simulink library "libbha_bha"  (R2015b)
settings: Solver=FixedStepDiscrete  StartTime=0.0  StopTime=Inf  FixedStep=0.004  RelTol=1e-3
PostLoadFcn:
  | , if any(exist('dsrtsu_mdlpostloadfcn', 'file') == [2, 3, 6]), try dsrtsu_mdlpostloadfcn('Execute', bdroot); catch fprintf('Error in PostLoadFcn (dsrtsu_mdlpostloadfcn) for model "%s":\n %s\n', bdroot, lasterr); end, end,
undefined symbols (not defined in the file or in its folder): accurate, BHA, O
libraries: libbha_io x7, libc_filters_diff x6, libbha_kinematic_tools x6, rtilibm x4, libbha_bha x1, libc_extended_basics x1
settings Model: DSRTSU_INTERNAL_RTI_VER=470  DSRTSU_INTERNAL_RTI_TYPE=rti1007  DSRTSU_INTERNAL_RTIFPGA=60  Creator=Falkenhahn  LastModifiedBy=isysfalkenhahn
settings DataIOCC: SaveFormat=Array
settings OptimizationCC: BlockReduction=off  OptimizeBlockIOStorage=off  BufferReuse=off  GlobalBufferReuse=off  ExpressionFolding=off  LocalBlockOutputs=off
settings DebuggingCC: UnderspecifiedInitializationDetection=Classic  MergeDetectMultiDrivingBlocksExec=none  SolverPrmCheckMsg=warning
settings HardwareCC: ProdBitPerPointer=32  ProdLargestAtomicFloat=None  ProdEndianess=BigEndian  ProdWordSize=32  ProdHWDeviceType=Generic->Custom  TargetIntDivRoundTo=Zero  TargetEndianess=BigEndian  TargetHWDeviceType=Generic->Custom
settings RTWCC: SystemTargetFile=rti1007.tlc  MakeCommand=make_rti  TemplateMakefile=rti1007.tmf  Description=dSPACE DS1007 Hardware Platform
settings STFCustomTargetCC: ParMdlRefBuildCompliant=on  ConcurrentExecutionCompliant=off  MatFileLogging=on  SystemTargetFile=rti1007.tlc
settings GRTTargetCC: CompOptLevelCompliant=off  ConcurrentExecutionCompliant=off  GeneratePreprocessorConditionals=Disable all  CombineOutputUpdateFcns=off  GRTInterface=on  UseToolchainInfoCompliant=off  ExtModeMexFile=noextcomm
settings ConfigComp: CovModelRefEnable=Off

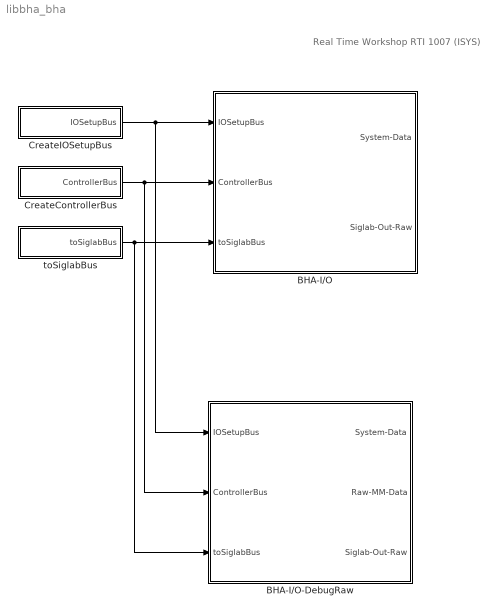
== system libbha_bha ==
  note: Real Time Workshop
      | RTI 1007 (ISYS)
  BHA-I/O : Subsystem  mask{tA=0.001 % CONST.tA, tA_mm=0.001 % CTRL.Measurement.tA, tA_mm_CAN=0.001 % CTRL.Measurement.tA_CAN, f_length=24 % CTRL.Measurement.f_filt_length, f_pressure=25 % 50 % CTRL.Measurement.f_filt_pressure, f_raw=0.1 % CTRL.Measurement.f_filt_raw}
      mask prompts: tA "simulation sample time [s]"; tA_mm "measurement sample time [s]"; tA_mm_CAN "measurement sample time (CAN) [s]"; f_length "filter frequency length [Hz]"; f_pressure "filter frequency pressure [Hz]"; f_raw "filter frequency raw [Hz]"
      settings: AttributesFormatString=|
      | simulation sample time: %<tA>
      | mm sample time: %<tA_mm>
      | mm sample time (CAN): %<tA_mm_CAN>
      | filter length: %<f_length> Hz
      | filter pressure: %<f_pressure> Hz
      | filter raw: %<f_raw> Hz
  BHA-I/O-DebugRaw : Subsystem  mask{tA=0.001 % CONST.tA, tA_mm=0.001 % CTRL.Measurement.tA, tA_mm_CAN=0.004 % CTRL.Measurement.tA_CAN, f_length=24 % CTRL.Measurement.f_filt_length, f_pressure=24 % 50 % CTRL.Measurement.f_filt_pressure, f_raw=0.1 % CTRL.Measurement.f_filt_raw}
      mask prompts: tA "simulation sample time [s]"; tA_mm "measurement sample time [s]"; tA_mm_CAN "measurement sample time (CAN) [s]"; f_length "filter frequency length [Hz]"; f_pressure "filter frequency pressure [Hz]"; f_raw "filter frequency raw [Hz]"
      settings: AttributesFormatString=|
      | simulation sample time: %<tA>
      | mm sample time: %<tA_mm>
      | mm sample time (CAN): %<tA_mm_CAN>
      | filter length: %<f_length> Hz
      | filter pressure: %<f_pressure> Hz
      | filter raw: %<f_raw> Hz
  CreateControllerBus : Subsystem
  CreateIOSetupBus : Subsystem
  toSiglabBus : Subsystem
  wires:
  CreateIOSetupBus/1(IOSetupBus) -> BHA-I/O/1(IOSetupBus), BHA-I/O-DebugRaw/1(IOSetupBus)
  CreateControllerBus/1(ControllerBus) -> BHA-I/O/2(ControllerBus), BHA-I/O-DebugRaw/2(ControllerBus)
  toSiglabBus/1(toSiglabBus) -> BHA-I/O/3(toSiglabBus), BHA-I/O-DebugRaw/3(toSiglabBus)

== system libbha_bha/BHA-I//O ==
  note: Real Time Workshop
      | RTI 1007 (ISYS)
  IOSetupBus : Inport
  ControllerBus : Inport  Port=2
  toSiglabBus : Inport  Port=3
  BHA-I/O-DebugRaw : libbha_bha/BHA-I//O-DebugRaw  tA=tA  tA_mm=tA_mm  tA_mm_CAN=tA_mm_CAN  f_length=f_length  f_pressure=f_pressure  f_raw=f_raw
      settings: AttributesFormatString=|
      | simulation sample time: %<tA>
      | mm sample time: %<tA_mm>
      | mm sample time (CAN): %<tA_mm_CAN>
      | filter length: %<f_length> Hz
      | filter pressure: %<f_pressure> Hz
      | filter raw: %<f_raw> Hz
  Terminator : Terminator
  System-Data : Outport
  Siglab-Out-Raw : Outport  Port=2
  wires:
  BHA-I/O-DebugRaw/1 -> System-Data/1
  BHA-I/O-DebugRaw/3 -> Siglab-Out-Raw/1
  toSiglabBus/1 -> BHA-I/O-DebugRaw/3
  ControllerBus/1 -> BHA-I/O-DebugRaw/2
  IOSetupBus/1 -> BHA-I/O-DebugRaw/1
  BHA-I/O-DebugRaw/2 -> Terminator/1

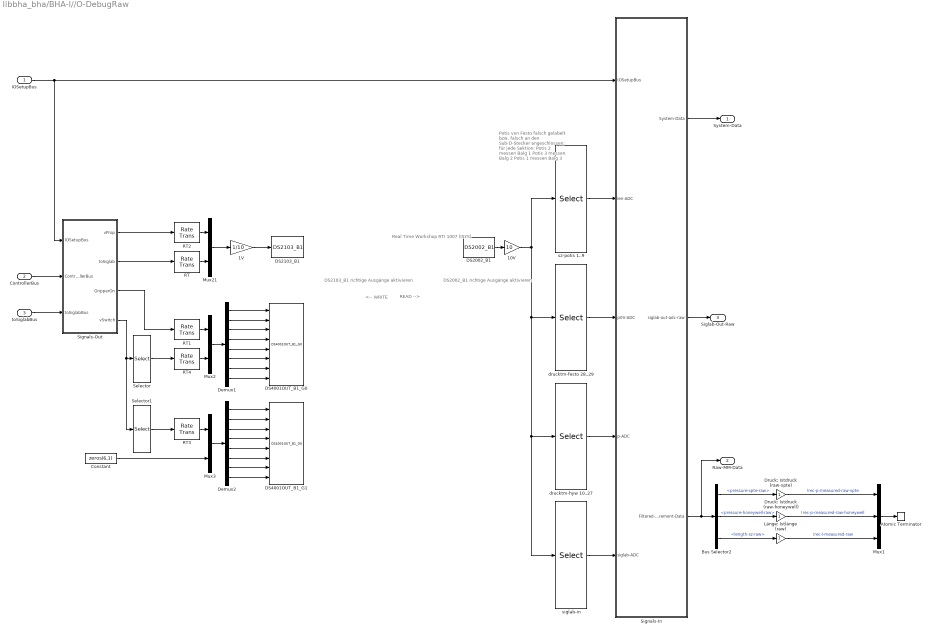
== system libbha_bha/BHA-I//O-DebugRaw ==
  note: Potis von Festo falsch
      | gelabelt bzw. falsch an
      | den Sub-D-Stecker
      | angeschlossen:
      | für jede Sektion:
      | Potis 2 messen Balg 1
      | Potis 3 messen Balg 2
      | Potis 1 messen Balg 3
  note: DS2103_B1 richtige Ausgänge aktivieren
  note: DS2002_B1 richtige Ausgänge aktivieren
  note: <-- WRITE
  note: READ -->
  note: Real Time Workshop
      | RTI 1007 (ISYS)
  IOSetupBus : Inport
  ControllerBus : Inport  Port=2
  toSiglabBus : Inport  Port=3
  10V : Gain  Gain=10
  1V : Gain  Gain=1/10
  Atomic Terminator : libc_extended_basics/Atomic Terminator
  Bus Selector2 : BusSelector  OutputSignals=pressure-spte-raw,pressure-honeywell-raw,length-sz-raw
  Constant : Constant  Value=zeros(6,1)  OutDataTypeStr=boolean
  DS2002_B1 : rtilibm/DS2002/DS2002_B1  BoardNo=1  ChannelNos=[1 2 3 4 5 6 7 8 9 10 11 12 13 14 15 16 17 18 19 20 21 22 23 24 25 26 27 28 29 30 31 32]  Range=[10 10]  Resolution=[16 16]  SampleAndHoldMode=[1 1]  DialogFcn=gui2002  UnitName={ 'DS2002_B' }  UnitValues={ 1 }  DSProperties=struct('RTI',struct('Version',uint32(1),'BlockType',struct('isSLSource',uint8(1),'isSLSink',uint8(0),'isHWSource',uint8(1),'isHWSink',uint8(0),'isSetup',uint8(0),'isInline',uint8(1),'isNonInline',uint8(0),'isInterrupt',uint8(0),'isChannelwise',uint8(0)),'IOBoardType','DS2002','UnitType','ADC','Identifier','ADCMUX','DialogType','ML','BlockSet','NONE','SlaveProcessor','NONE'))
  DS2103_B1 : rtilibm/DS2103/DS2103_B1  BoardNo=1  ChannelNos=[1 2 3 4 5 6 7 8 9 10 11 12]  Range=[10 10 10 10 10 10 10 10 10 10 10 10 10 10 10 10 10 10 10 10 10 10 10 10 10 10 10 10 10 10 10 10]  IOErrorMode=[1 1 1 1 1 1 1 1]  InitValue=[0.5 0.5 0.5 0.5 0.5 0.5 0.5 0.5 0 0 0 0 0 0 0 0 0 0 0 0 0 0 0 0 0 0 0 0 0 0 0 0]  TermMode=[0 0 0 0 0 0 0 0 1 1 1 1 1 1 1 1 1 1 1 1 1 1 1 1 1 1 1 1 1 1 1 1]  TermValue=[0 0 0 0 0 0 0 0 0 0 0 0 0 0 0 0 0 0 0 0 0 0 0 0 0 0 0 0 0 0 0 0]  DialogFcn=gui2103  UnitName={ 'DS2103_B' }  UnitValues={ 1 }  DSProperties=struct('RTI',struct('Version',uint32(1),'BlockType',struct('isSLSource',uint8(0),'isSLSink',uint8(1),'isHWSource',uint8(0),'isHWSink',uint8(1),'isSetup',uint8(0),'isInline',uint8(1),'isNonInline',uint8(0),'isInterrupt',uint8(0),'isChannelwise',uint8(0)),'IOBoardType','DS2103','UnitType','DAC','Identifier','DACMUX','DialogType','ML','BlockSet','NONE','SlaveProcessor','NONE'))
  DS4001OUT_B1_G0 : rtilibm/DS4001/DS4001OUT_B1_G0  BoardNo=1  GroupNo=0  InitValue=[0 0 0 0 0 0 0 0]  TermMode=[1 1 1 1 1 1 1 1]  TermValue=[0 0 0 0 0 0 0 0]  DialogFcn=gui400xout  UnitName={ 'DS4001OUT_B', '_G' }  UnitValues="{ 1  0 }"  DSProperties=struct('RTI',struct('Version',uint32(1),'BlockType',struct('isSLSource',uint8(0),'isSLSink',uint8(1),'isHWSource',uint8(0),'isHWSink',uint8(1),'isSetup',uint8(0),'isInline',uint8(1),'isNonInline',uint8(0),'isInterrupt',uint8(0),'isChannelwise',uint8(0)),'IOBoardType','DS4001','UnitType','BIT','Identifier','BITOUT','DialogType','ML','BlockSet','NONE','SlaveProcessor','NONE'))
  DS4001OUT_B1_G1 : rtilibm/DS4001/DS4001OUT_B1_G0  BoardNo=1  GroupNo=1  InitValue=[0 0 0 0 0 0 0 0]  TermMode=[1 1 1 1 1 1 1 1]  TermValue=[0 0 0 0 0 0 0 0]  DialogFcn=gui400xout  UnitName={ 'DS4001OUT_B', '_G' }  UnitValues="{1  1}"  DSProperties=struct('RTI',struct('Version',uint32(1),'BlockType',struct('isSLSource',uint8(0),'isSLSink',uint8(1),'isHWSource',uint8(0),'isHWSink',uint8(1),'isSetup',uint8(0),'isInline',uint8(1),'isNonInline',uint8(0),'isInterrupt',uint8(0),'isChannelwise',uint8(0)),'IOBoardType','DS4001','UnitType','BIT','Identifier','BITOUT','DialogType','ML','BlockSet','NONE','SlaveProcessor','NONE'))
  Demux1 : Demux  Outputs=8
  Demux2 : Demux  Outputs=8
  Druck: Istdruck (raw-honeywell) : Gain
  Druck: Istdruck (raw-spte) : Gain
  Länge: Istlänge (raw) : Gain
  Mux1 : Mux  Inputs=3
  Mux2 : Mux  Inputs=2
  Mux21 : Mux  Inputs=2
  Mux3 : Mux  Inputs=2
  RT{,1..4} (5 alike) : RateTransition  Deterministic=off  OutPortSampleTime=tA_mm
  Selector : Selector  InputPortWidth=9  IndexOptions=Index vector (dialog)  Indices=[1 2 3 4 5 6 7]  OutputSizes=1
  Selector1 : Selector  InputPortWidth=9  IndexOptions=Index vector (dialog)  Indices=[8 9]  OutputSizes=1
  Signals-In : Subsystem
      settings: AttributesFormatString=|
      | sample time: tA
      | (simulation sample time)
  Signals-Out : Subsystem
  drucktm-festo 28..29 : Selector  InputPortWidth=32  IndexOptions=Index vector (dialog)  Indices=[28 29]  OutputSizes=1
  "drucktm-hyw 10..27 " : Selector  InputPortWidth=32  IndexOptions=Index vector (dialog)  Indices=[10 11 12 13 14 15 16 17 18 19 20 21 22 23 24 25 26 27]  OutputSizes=1
  siglab-in : Selector  InputPortWidth=32  IndexOptions=Index vector (dialog)  Indices=[30 31 32]  OutputSizes=1
  sz-potis 1..9 : Selector  InputPortWidth=32  IndexOptions=Index vector (dialog)  Indices=[2 3 1 5 6 4 8 9 7]  OutputSizes=1
  System-Data : Outport
  Raw-MM-Data : Outport  Port=2
  Siglab-Out-Raw : Outport  Port=3
  wires:
  RT3/1 -> Mux3/1
  Mux3/1 -> Demux2/1
  RT4/1 -> Mux2/2
  RT1/1 -> Mux2/1
  Mux2/1 -> Demux1/1
  Bus Selector2/2 -> Druck: Istdruck (raw-honeywell)/1  "<pressure-honeywell-raw>"
  Bus Selector2/3 -> Länge: Istlänge (raw)/1  "<length-sz-raw>"
  Druck: Istdruck (raw-honeywell)/1 -> Mux1/2  "!rec-p-measured-raw-honeywell"
  Länge: Istlänge (raw)/1 -> Mux1/3  "!rec-l-measured-raw"
  Mux1/1 -> Atomic Terminator/1
  Signals-In/1(System-Data) -> System-Data/1
  toSiglabBus/1 -> Signals-Out/3(toSiglabBus)
  IOSetupBus/1 -> Signals-In/1(IOSetupBus), Signals-Out/1(IOSetupBus)
  ControllerBus/1 -> Signals-Out/2(ControllerBus)
  Signals-Out/2(toSiglab) -> RT/1
  Signals-Out/1(vProp) -> RT2/1
  1V/1 -> DS2103_B1/1
  10V/1 -> siglab-in/1, "drucktm-hyw 10..27 "/1, drucktm-festo 28..29/1, sz-potis 1..9/1
  DS2002_B1/1 -> 10V/1
  Mux21/1 -> 1V/1
  RT2/1 -> Mux21/1
  RT/1 -> Mux21/2
  Demux1/2 -> DS4001OUT_B1_G0/2
  Demux1/6 -> DS4001OUT_B1_G0/6
  Demux1/1 -> DS4001OUT_B1_G0/1
  Demux1/3 -> DS4001OUT_B1_G0/3
  Demux1/5 -> DS4001OUT_B1_G0/5
  Demux1/8 -> DS4001OUT_B1_G0/8
  Demux1/4 -> DS4001OUT_B1_G0/4
  Demux1/7 -> DS4001OUT_B1_G0/7
  Demux2/3 -> DS4001OUT_B1_G1/3
  Demux2/1 -> DS4001OUT_B1_G1/1
  Demux2/4 -> DS4001OUT_B1_G1/4
  Demux2/2 -> DS4001OUT_B1_G1/2
  Demux2/5 -> DS4001OUT_B1_G1/5
  Demux2/6 -> DS4001OUT_B1_G1/6
  Demux2/7 -> DS4001OUT_B1_G1/7
  Demux2/8 -> DS4001OUT_B1_G1/8
  Signals-Out/4(vSwitch) -> Selector1/1, Selector/1
  Signals-Out/3(GripperOn) -> RT1/1
  Selector/1 -> RT4/1
  Selector1/1 -> RT3/1
  Constant/1 -> Mux3/2
  sz-potis 1..9/1 -> Signals-In/2(len-ADC)
  drucktm-festo 28..29/1 -> Signals-In/3(p0V-ADC)
  siglab-in/1 -> Signals-In/5(siglab-ADC)
  "drucktm-hyw 10..27 "/1 -> Signals-In/4(p-ADC)
  Signals-In/3(Filtered-Raw-Measurement-Data) -> Bus Selector2/1, Raw-MM-Data/1
  Signals-In/2(siglab-out-adc-raw) -> Siglab-Out-Raw/1
  Bus Selector2/1 -> Druck: Istdruck (raw-spte)/1  "<pressure-spte-raw>"
  Druck: Istdruck (raw-spte)/1 -> Mux1/1  "!rec-p-measured-raw-spte"

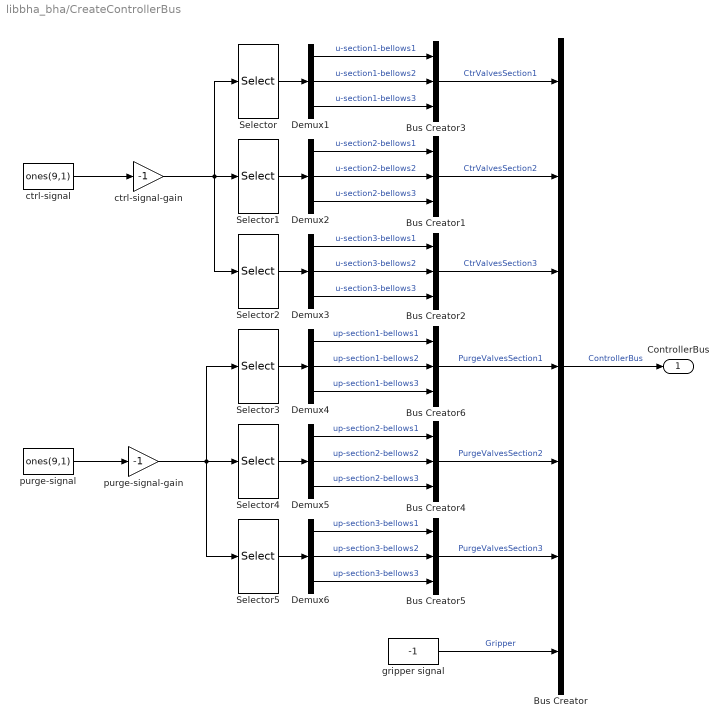
== system libbha_bha/CreateControllerBus ==
  Bus Creator : BusCreator  Inputs=7
  Bus Creator{1..6} (6 alike) : BusCreator  Inputs=3
  Demux{1..6} (6 alike) : Demux  Outputs=3
  Selector : Selector  InputPortWidth=9  IndexOptions=Index vector (dialog)  Indices=[1 2 3]  OutputSizes=1
  Selector1 : Selector  InputPortWidth=9  IndexOptions=Index vector (dialog)  Indices=[4 5 6]  OutputSizes=1
  Selector2 : Selector  InputPortWidth=9  IndexOptions=Index vector (dialog)  Indices=[7 8 9]  OutputSizes=1
  Selector3 : Selector  InputPortWidth=9  IndexOptions=Index vector (dialog)  Indices=[1 2 3]  OutputSizes=1
  Selector4 : Selector  InputPortWidth=9  IndexOptions=Index vector (dialog)  Indices=[4 5 6]  OutputSizes=1
  Selector5 : Selector  InputPortWidth=9  IndexOptions=Index vector (dialog)  Indices=[7 8 9]  OutputSizes=1
  ctrl-signal : Constant  Value=ones(9,1)
  ctrl-signal-gain : Gain  Gain=-1
  gripper signal : Constant  Value=-1
  purge-signal : Constant  Value=ones(9,1)
  purge-signal-gain : Gain  Gain=-1
  ControllerBus : Outport
  wires:
  Demux3/3 -> Bus Creator2/3  "u-section3-bellows3"
  Demux3/2 -> Bus Creator2/2  "u-section3-bellows2"
  Demux3/1 -> Bus Creator2/1  "u-section3-bellows1"
  Demux2/1 -> Bus Creator1/1  "u-section2-bellows1"
  Demux2/2 -> Bus Creator1/2  "u-section2-bellows2"
  Demux2/3 -> Bus Creator1/3  "u-section2-bellows3"
  Demux1/1 -> Bus Creator3/1  "u-section1-bellows1"
  Demux1/2 -> Bus Creator3/2  "u-section1-bellows2"
  Demux1/3 -> Bus Creator3/3  "u-section1-bellows3"
  Bus Creator/1 -> ControllerBus/1  "ControllerBus"
  Selector/1 -> Demux1/1
  Selector1/1 -> Demux2/1
  Selector2/1 -> Demux3/1
  Bus Creator3/1 -> Bus Creator/1  "CtrValvesSection1"
  Bus Creator1/1 -> Bus Creator/2  "CtrValvesSection2"
  Bus Creator2/1 -> Bus Creator/3  "CtrValvesSection3"
  Demux6/3 -> Bus Creator5/3  "up-section3-bellows3"
  Demux6/2 -> Bus Creator5/2  "up-section3-bellows2"
  Demux6/1 -> Bus Creator5/1  "up-section3-bellows1"
  Demux5/1 -> Bus Creator4/1  "up-section2-bellows1"
  Demux5/2 -> Bus Creator4/2  "up-section2-bellows2"
  Demux5/3 -> Bus Creator4/3  "up-section2-bellows3"
  Demux4/1 -> Bus Creator6/1  "up-section1-bellows1"
  Demux4/2 -> Bus Creator6/2  "up-section1-bellows2"
  Demux4/3 -> Bus Creator6/3  "up-section1-bellows3"
  Selector3/1 -> Demux4/1
  Selector4/1 -> Demux5/1
  Selector5/1 -> Demux6/1
  Bus Creator6/1 -> Bus Creator/4  "PurgeValvesSection1"
  Bus Creator4/1 -> Bus Creator/5  "PurgeValvesSection2"
  Bus Creator5/1 -> Bus Creator/6  "PurgeValvesSection3"
  ctrl-signal/1 -> ctrl-signal-gain/1
  purge-signal/1 -> purge-signal-gain/1
  purge-signal-gain/1 -> Selector5/1, Selector3/1, Selector4/1
  ctrl-signal-gain/1 -> Selector2/1, Selector/1, Selector1/1
  gripper signal/1 -> Bus Creator/7  "Gripper"

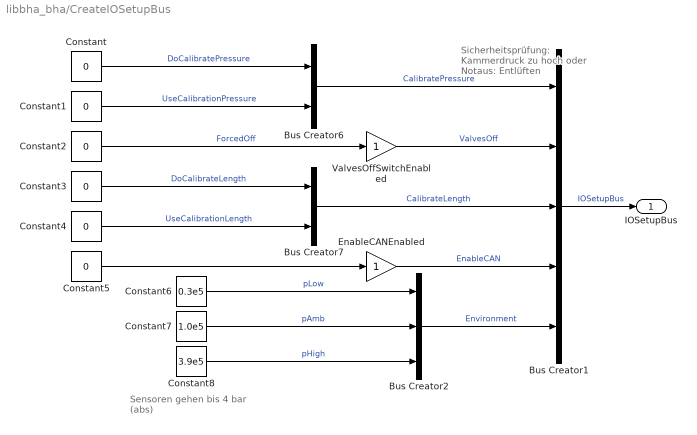
== system libbha_bha/CreateIOSetupBus ==
  note: Sensoren gehen bis 4 bar (abs)
  note: Sicherheitsprüfung:
      | Kammerdruck zu hoch
      | oder Notaus: Entlüften
  Bus Creator1 : BusCreator  Inputs=5
  Bus Creator2 : BusCreator  Inputs=3
  Bus Creator6 : BusCreator  Inputs=2
  Bus Creator7 : BusCreator  Inputs=2
  Constant{,1..5} (6 alike) : Constant  Value=0
  Constant6 : Constant  Value=0.3e5
  Constant7 : Constant  Value=1.0e5
  Constant8 : Constant  Value=3.9e5
  EnableCANEnabled : Gain
  ValvesOffSwitchEnabled : Gain
  IOSetupBus : Outport
  wires:
  Constant8/1 -> Bus Creator2/3  "pHigh"
  Constant7/1 -> Bus Creator2/2  "pAmb"
  Constant6/1 -> Bus Creator2/1  "pLow"
  Bus Creator1/1 -> IOSetupBus/1  "IOSetupBus"
  Bus Creator7/1 -> Bus Creator1/3  "CalibrateLength"
  Constant/1 -> Bus Creator6/1  "DoCalibratePressure"
  Constant1/1 -> Bus Creator6/2  "UseCalibrationPressure"
  Constant3/1 -> Bus Creator7/1  "DoCalibrateLength"
  Constant4/1 -> Bus Creator7/2  "UseCalibrationLength"
  Bus Creator2/1 -> Bus Creator1/5  "Environment"
  ValvesOffSwitchEnabled/1 -> Bus Creator1/2  "ValvesOff"
  Bus Creator6/1 -> Bus Creator1/1  "CalibratePressure"
  Constant5/1 -> EnableCANEnabled/1
  EnableCANEnabled/1 -> Bus Creator1/4  "EnableCAN"
  Constant2/1 -> ValvesOffSwitchEnabled/1  "ForcedOff"

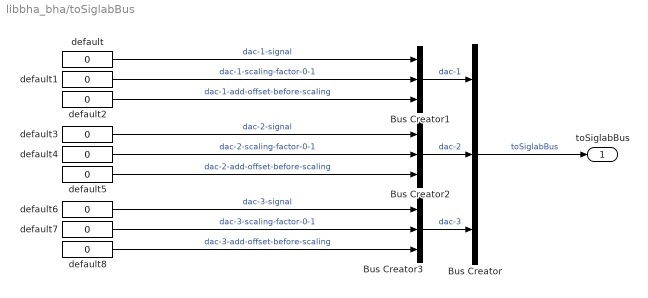
== system libbha_bha/toSiglabBus ==
  Bus Creator{,1..3} (4 alike) : BusCreator  Inputs=3
  default{,1..8} (9 alike) : Constant  Value=0
  toSiglabBus : Outport
  wires:
  default6/1 -> Bus Creator3/1  "dac-3-signal"
  default7/1 -> Bus Creator3/2  "dac-3-scaling-factor-0-1"
  default8/1 -> Bus Creator3/3  "dac-3-add-offset-before-scaling"
  default3/1 -> Bus Creator2/1  "dac-2-signal"
  default4/1 -> Bus Creator2/2  "dac-2-scaling-factor-0-1"
  default5/1 -> Bus Creator2/3  "dac-2-add-offset-before-scaling"
  default2/1 -> Bus Creator1/3  "dac-1-add-offset-before-scaling"
  default/1 -> Bus Creator1/1  "dac-1-signal"
  default1/1 -> Bus Creator1/2  "dac-1-scaling-factor-0-1"
  Bus Creator3/1 -> Bus Creator/3  "dac-3"
  Bus Creator2/1 -> Bus Creator/2  "dac-2"
  Bus Creator1/1 -> Bus Creator/1  "dac-1"
  Bus Creator/1 -> toSiglabBus/1  "toSiglabBus"

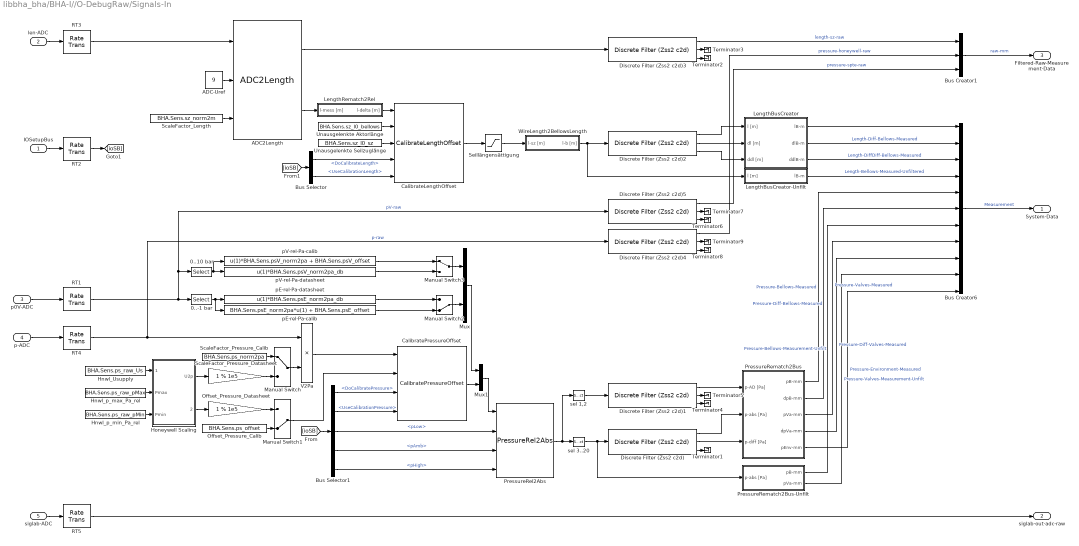
== system libbha_bha/BHA-I//O-DebugRaw/Signals-In ==
  IOSetupBus : Inport
  len-ADC : Inport  Port=2
  p0V-ADC : Inport  Port=3
  p-ADC : Inport  Port=4
      settings: AttributesFormatString=|
      | 1..9 pValves (a)
      | 10..18 pBellows (b)
  siglab-ADC : Inport  Port=5
  0..-1 bar : Selector  InputPortWidth=2  IndexOptions=Index vector (dialog)  Indices=1  OutputSizes=1
      settings: AttributesFormatString=0..10 V
  0..10 bar : Selector  InputPortWidth=2  IndexOptions=Index vector (dialog)  Indices=2  OutputSizes=1
      settings: AttributesFormatString=0..10 V
  ADC-Uref : Constant  Value=9
  ADC2Length : libbha_io/ADC2Length
  Bus Creator1 : BusCreator  Inputs=3
  Bus Creator6 : BusCreator  Inputs=11
  Bus Selector : BusSelector  OutputSignals=CalibrateLength.DoCalibrateLength,CalibrateLength.UseCalibrationLength
  Bus Selector1 : BusSelector  OutputSignals=CalibratePressure.DoCalibratePressure,CalibratePressure.UseCalibrationPressure,Environment.pLow,Environment.pAmb,Environment.pHigh
  CalibrateLengthOffset : libbha_io/CalibrateLengthOffset
  CalibratePressureOffset : libbha_io/CalibratePressureOffset
      settings: AttributesFormatString=Dimension: %<dim>
  Discrete Filter (Zss2 c2d) : libc_filters_diff/Discrete Filter (Zss2 c2d)  rdnname2342_gf=f_pressure  rdnname2342_tA=tA  rdnname2342_mode=noh (d=0)  rdnname2342_diffmode=O(2) [accurate]  rdnname2342_showd=on
      settings: AttributesFormatString=%<rdnname2342_gf> Hz, %<rdnname2342_mode>
  Discrete Filter (Zss2 c2d)1 : libc_filters_diff/Discrete Filter (Zss2 c2d)  rdnname2342_gf=f_pressure  rdnname2342_tA=tA  rdnname2342_mode=noh (d=0)  rdnname2342_diffmode=O(2) [accurate]  rdnname2342_showd=on
      settings: AttributesFormatString=%<rdnname2342_gf> Hz, %<rdnname2342_mode>
  Discrete Filter (Zss2 c2d)2 : libc_filters_diff/Discrete Filter (Zss2 c2d)  rdnname2342_gf=f_length  rdnname2342_tA=tA  rdnname2342_mode=noh (d=0)  rdnname2342_diffmode=O(2) [accurate]  rdnname2342_showd=on
      settings: AttributesFormatString=%<rdnname2342_gf> Hz, %<rdnname2342_mode>
  Discrete Filter (Zss2 c2d)3 : libc_filters_diff/Discrete Filter (Zss2 c2d)  rdnname2342_gf=f_raw  rdnname2342_tA=tA  rdnname2342_mode=zoh (d=dt)  rdnname2342_diffmode=O(2) [accurate]  rdnname2342_showd=on
      settings: AttributesFormatString=%<rdnname2342_gf> Hz, %<rdnname2342_mode>
  Discrete Filter (Zss2 c2d)4 : libc_filters_diff/Discrete Filter (Zss2 c2d)  rdnname2342_gf=f_raw  rdnname2342_tA=tA  rdnname2342_mode=zoh (d=dt)  rdnname2342_diffmode=O(2) [accurate]  rdnname2342_showd=on
      settings: AttributesFormatString=%<rdnname2342_gf> Hz, %<rdnname2342_mode>
  Discrete Filter (Zss2 c2d)5 : libc_filters_diff/Discrete Filter (Zss2 c2d)  rdnname2342_gf=f_raw  rdnname2342_tA=tA  rdnname2342_mode=zoh (d=dt)  rdnname2342_diffmode=O(2) [accurate]  rdnname2342_showd=on
      settings: AttributesFormatString=%<rdnname2342_gf> Hz, %<rdnname2342_mode>
  Hnwl_Usupply : Constant  Value=BHA.Sens.ps_raw_Us
  Hnwl_p_max_Pa_rel : Constant  Value=BHA.Sens.ps_raw_pMax
  Hnwl_p_min_Pa_rel : Constant  Value=BHA.Sens.ps_raw_pMin
  Honeywell Scaling : MATLAB Function  TreatAsAtomicUnit=on
  LengthBusCreator : Subsystem
  LengthBusCreator-Unfilt : Subsystem
  LengthRematch2Rel : Subsystem
  Manual Switch : ManualSwitch
  Manual Switch1 : ManualSwitch  CurrentSetting=0
  Manual Switch2 : ManualSwitch  CurrentSetting=0
  Manual Switch3 : ManualSwitch
  Mux : Mux  Inputs=2
  Mux1 : Mux  Inputs=2
  Offset_Pressure_Calib : Constant  Value=BHA.Sens.ps_offset
  Offset_Pressure_Datasheet : Gain  Gain=1 % 1e5
  PressureRel2Abs : libbha_io/PressureRel2Abs
  PressureRematch2Bus : Subsystem
  PressureRematch2Bus-Unfilt : Subsystem
  RT1 : RateTransition  Deterministic=off  X0=1.1  OutPortSampleTime=tA
      settings: AttributesFormatString=|
      | sinnv. Anfangswert:
      | 1.1
  RT2 : RateTransition  Deterministic=off  OutPortSampleTime=tA
  RT3 : RateTransition  Deterministic=off  X0=[3 3 3 4 4 4 5 5 5]  OutPortSampleTime=tA
      settings: AttributesFormatString=|
      | sinnv. Anfangswerte:
      | [ 3 3 3 4 4 4 5 5 5 ]
  RT4 : RateTransition  Deterministic=off  X0=5  OutPortSampleTime=tA
      settings: AttributesFormatString=|
      | sinnv. Anfangswert:
      | 5
  RT5 : RateTransition  Deterministic=off  OutPortSampleTime=tA
  ScaleFactor_Length : Constant  Value=BHA.Sens.sz_norm2m
  ScaleFactor_Pressure_Calib : Constant  Value=BHA.Sens.ps_norm2pa
  ScaleFactor_Pressure_Datasheet : Gain  Gain=1 % 1e5
  Seillängensättigung : Saturate  UpperLimit=2.0  LowerLimit=0.1
      settings: AttributesFormatString=0.1 bis 2.0
  Terminator{1..9} (9 alike) : Terminator
  Unausgelenkte Aktorlänge : Constant  Value=BHA.Sens.sz_l0_bellows
  Unausgelenkte Seilzuglänge : Constant  Value=BHA.Sens.sz_l0_sz
  V2Pa : Product
  WireLength2BellowsLength : Subsystem
  pE-rel-Pa-calib : Fcn  Expr=BHA.Sens.psE_norm2pa*u(1) + BHA.Sens.psE_offset
  pE-rel-Pa-datasheet : Fcn  Expr=u(1)*BHA.Sens.psE_norm2pa_db
  pV-rel-Pa-calib : Fcn  Expr=u(1)*BHA.Sens.psV_norm2pa + BHA.Sens.psV_offset
  pV-rel-Pa-datasheet : Fcn  Expr=u(1)*BHA.Sens.psV_norm2pa_db
  sel 1,2 : Selector  InputPortWidth=20  IndexOptions=Index vector (dialog)  Indices=[1 2]  OutputSizes=1
  sel 3..20 : Selector  InputPortWidth=20  IndexOptions=Starting index (dialog)  Indices=3  OutputSizes=18
  System-Data : Outport
  siglab-out-adc-raw : Outport  Port=2
  Filtered-Raw-Measurement-Data : Outport  Port=3
  wires:
  Offset_Pressure_Calib/1 -> Manual Switch1/2
  ScaleFactor_Pressure_Calib/1 -> Manual Switch/1
  Offset_Pressure_Datasheet/1 -> Manual Switch1/1
  ScaleFactor_Pressure_Datasheet/1 -> Manual Switch/2
  pE-rel-Pa-datasheet/1 -> Manual Switch2/1
  pV-rel-Pa-datasheet/1 -> Manual Switch3/2
  0..-1 bar/1 -> pE-rel-Pa-calib/1, pE-rel-Pa-datasheet/1
  0..10 bar/1 -> pV-rel-Pa-calib/1, pV-rel-Pa-datasheet/1
  Manual Switch1/1 -> CalibratePressureOffset/2
  Manual Switch/1 -> V2Pa/2
  Honeywell Scaling/2(offset_p) -> Offset_Pressure_Datasheet/1
  Honeywell Scaling/1(U2p) -> ScaleFactor_Pressure_Datasheet/1
  Hnwl_p_min_Pa_rel/1 -> Honeywell Scaling/3(Pmin)
  Hnwl_p_max_Pa_rel/1 -> Honeywell Scaling/2(Pmax)
  Hnwl_Usupply/1 -> Honeywell Scaling/1(Vsupply)
  Bus Creator1/1 -> Filtered-Raw-Measurement-Data/1  "raw-mm"
  Discrete Filter (Zss2 c2d)4/1 -> Bus Creator1/2  "pressure-honeywell-raw"
  Discrete Filter (Zss2 c2d)5/1 -> Bus Creator1/3  "pressure-spte-raw"
  Discrete Filter (Zss2 c2d)4/3 -> Terminator8/1
  Discrete Filter (Zss2 c2d)4/2 -> Terminator9/1
  Discrete Filter (Zss2 c2d)5/3 -> Terminator6/1
  Discrete Filter (Zss2 c2d)5/2 -> Terminator7/1
  Discrete Filter (Zss2 c2d)3/3 -> Terminator2/1
  Discrete Filter (Zss2 c2d)3/2 -> Terminator3/1
  Discrete Filter (Zss2 c2d)3/1 -> Bus Creator1/1  "length-sz-raw"
  PressureRematch2Bus/4(dpVa-mm) -> Bus Creator6/9  "Pressure-Diff-Valves-Measured"
  PressureRematch2Bus/3(pVa-mm) -> Bus Creator6/8  "Pressure-Valves-Measured"
  PressureRematch2Bus-Unfilt/2(pVa-mm) -> Bus Creator6/10  "Pressure-Valves-Measurement-Unfilt"
  LengthBusCreator/1(lB-m) -> Bus Creator6/1
  PressureRematch2Bus-Unfilt/1(pB-mm) -> Bus Creator6/7  "Pressure-Bellows-Measurement-Unfilt"
  LengthBusCreator-Unfilt/1(lB-m) -> Bus Creator6/4  "Length-Bellows-Measured-Unfiltered"
  LengthBusCreator/3(ddlB-m) -> Bus Creator6/3  "Length-DiffDiff-Bellows-Measured"
  LengthBusCreator/2(dlB-m) -> Bus Creator6/2  "Length-Diff-Bellows-Measured"
  PressureRematch2Bus/2(dpB-mm) -> Bus Creator6/6  "Pressure-Diff-Bellows-Measured"
  PressureRematch2Bus/5(pEnv-mm) -> Bus Creator6/11  "Pressure-Environment-Measured"
  PressureRematch2Bus/1(pB-mm) -> Bus Creator6/5  "Pressure-Bellows-Measured"
  Bus Creator6/1 -> System-Data/1  "Measurement"
  Discrete Filter (Zss2 c2d)1/1 -> PressureRematch2Bus/1(p-AD [Pa])
  Discrete Filter (Zss2 c2d)/1 -> PressureRematch2Bus/2(p-abs [Pa])
  Discrete Filter (Zss2 c2d)/2 -> PressureRematch2Bus/3(p-diff [Pa])
  Discrete Filter (Zss2 c2d)/3 -> Terminator1/1
  Discrete Filter (Zss2 c2d)1/3 -> Terminator4/1
  Discrete Filter (Zss2 c2d)1/2 -> Terminator5/1
  Discrete Filter (Zss2 c2d)2/3 -> LengthBusCreator/3(ddl [m])
  Discrete Filter (Zss2 c2d)2/2 -> LengthBusCreator/2(dl [m])
  Discrete Filter (Zss2 c2d)2/1 -> LengthBusCreator/1(l [m])
  sel 1,2/1 -> Discrete Filter (Zss2 c2d)1/1
  sel 3..20/1 -> Discrete Filter (Zss2 c2d)/1, PressureRematch2Bus-Unfilt/1(p-abs [Pa])
  RT5/1 -> siglab-out-adc-raw/1
  PressureRel2Abs/1 -> sel 1,2/1, sel 3..20/1
  WireLength2BellowsLength/1(l-b [m]) -> Discrete Filter (Zss2 c2d)2/1, LengthBusCreator-Unfilt/1(l [m])
  ScaleFactor_Length/1 -> ADC2Length/3
  CalibratePressureOffset/1 -> Mux1/2
  V2Pa/1 -> CalibratePressureOffset/1
  Bus Selector1/1 -> CalibratePressureOffset/3  "<DoCalibratePressure>"
  ADC2Length/1 -> Discrete Filter (Zss2 c2d)3/1
  RT4/1 -> V2Pa/1, Discrete Filter (Zss2 c2d)4/1  "p-raw"
  RT1/1 -> Discrete Filter (Zss2 c2d)5/1, 0..10 bar/1, 0..-1 bar/1  "pV-raw"
  RT3/1 -> ADC2Length/1
  ADC-Uref/1 -> ADC2Length/2
  RT2/1 -> [ioSB]
  siglab-ADC/1 -> RT5/1
  IOSetupBus/1 -> RT2/1
  Mux/1 -> Mux1/1
  p0V-ADC/1 -> RT1/1
  Mux1/1 -> PressureRel2Abs/1
  p-ADC/1 -> RT4/1
  Bus Selector1/5 -> PressureRel2Abs/4  "<pHigh>"
  Bus Selector1/4 -> PressureRel2Abs/3  "<pAmb>"
  Bus Selector1/3 -> PressureRel2Abs/2  "<pLow>"
  Bus Selector1/2 -> CalibratePressureOffset/4  "<UseCalibrationPressure>"
  [ioSB] -> Bus Selector1/1
  len-ADC/1 -> RT3/1
  Bus Selector/2 -> CalibrateLengthOffset/5  "<UseCalibrationLength>"
  Bus Selector/1 -> CalibrateLengthOffset/4  "<DoCalibrateLength>"
  [ioSB] -> Bus Selector/1
  pE-rel-Pa-calib/1 -> Manual Switch2/2
  pV-rel-Pa-calib/1 -> Manual Switch3/1
  Manual Switch3/1 -> Mux/1
  Manual Switch2/1 -> Mux/2
  ADC2Length/2 -> LengthRematch2Rel/1("l-mess [m] ")
  CalibrateLengthOffset/1 -> Seillängensättigung/1
  Unausgelenkte Seilzuglänge/1 -> CalibrateLengthOffset/3
  Unausgelenkte Aktorlänge/1 -> CalibrateLengthOffset/2
  LengthRematch2Rel/1(l-delta [m]) -> CalibrateLengthOffset/1
  Seillängensättigung/1 -> WireLength2BellowsLength/1(l-sz [m])

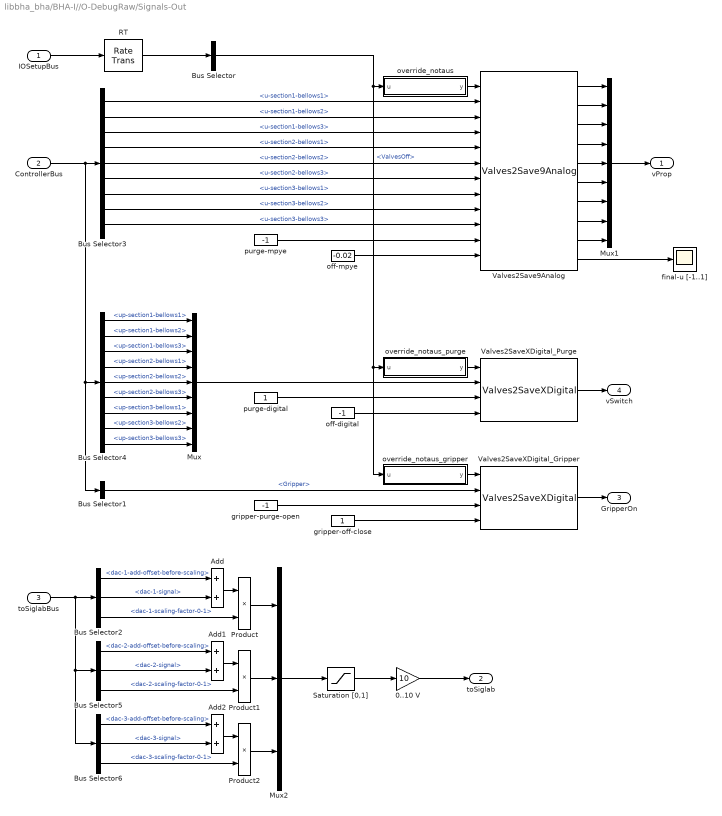
== system libbha_bha/BHA-I//O-DebugRaw/Signals-Out ==
  IOSetupBus : Inport
  ControllerBus : Inport  Port=2
  toSiglabBus : Inport  Port=3
  0..10 V : Gain  Gain=10
  Add : Sum
  Add1 : Sum
  Add2 : Sum
  Bus Selector : BusSelector  OutputSignals=ValvesOff
  Bus Selector1 : BusSelector  OutputSignals=Gripper
  Bus Selector2 : BusSelector  OutputSignals=dac-1.dac-1-add-offset-before-scaling,dac-1.dac-1-signal,dac-1.dac-1-scaling-factor-0-1
  Bus Selector3 : BusSelector  OutputSignals=CtrValvesSection1.u-section1-bellows1,CtrValvesSection1.u-section1-bellows2,CtrValvesSection1.u-section1-bellows3,CtrValvesSection2.u-section2-bellows1,CtrValvesSection2.u-section2-bellows2,CtrValvesSection2.u-section2-bellows3,CtrValvesSection3.u-section3-bellows1,CtrValvesSection3.u-section3-bellows2,CtrValvesSection3.u-section3-bellows3
  Bus Selector4 : BusSelector  OutputSignals=PurgeValvesSection1.up-section1-bellows1,PurgeValvesSection1.up-section1-bellows2,PurgeValvesSection1.up-section1-bellows3,PurgeValvesSection2.up-section2-bellows1,PurgeValvesSection2.up-section2-bellows2,PurgeValvesSection2.up-section2-bellows3,PurgeValvesSection3.up-section3-bellows1,PurgeValvesSection3.up-section3-bellows2,PurgeValvesSection3.up-section3-bellows3
  Bus Selector5 : BusSelector  OutputSignals=dac-2.dac-2-add-offset-before-scaling,dac-2.dac-2-signal,dac-2.dac-2-scaling-factor-0-1
  Bus Selector6 : BusSelector  OutputSignals=dac-3.dac-3-add-offset-before-scaling,dac-3.dac-3-signal,dac-3.dac-3-scaling-factor-0-1
  Mux : Mux  Inputs=9
  Mux1 : Mux  Inputs=9
  Mux2 : Mux  Inputs=3
  Product : Product
  Product1 : Product
  Product2 : Product
  RT : RateTransition  Deterministic=off
  Saturation [0,1] : Saturate  UpperLimit=1  LowerLimit=0
  Valves2Save9Analog : libbha_io/Valves2Save9Analog
  Valves2SaveXDigital_Gripper : libbha_io/Valves2SaveXDigital
  Valves2SaveXDigital_Purge : libbha_io/Valves2SaveXDigital
  final-u [-1..1] : Scope
  gripper-off-close : Constant
  gripper-purge-open : Constant  Value=-1
  off-digital : Constant  Value=-1
  off-mpye : Constant  Value=-0.02
  override_notaus : MATLAB Function  TreatAsAtomicUnit=on
  override_notaus_gripper : MATLAB Function  TreatAsAtomicUnit=on
  override_notaus_purge : MATLAB Function  TreatAsAtomicUnit=on
  purge-digital : Constant
  purge-mpye : Constant  Value=-1
  vProp : Outport
  toSiglab : Outport  Port=2
  GripperOn : Outport  Port=3
  vSwitch : Outport  Port=4
  wires:
  Add/1 -> Product/1
  Bus Selector2/3 -> Product/2  "<dac-1-scaling-factor-0-1>"
  Bus Selector2/2 -> Add/2  "<dac-1-signal>"
  Bus Selector2/1 -> Add/1  "<dac-1-add-offset-before-scaling>"
  0..10 V/1 -> toSiglab/1
  RT/1 -> Bus Selector/1
  Saturation [0,1]/1 -> 0..10 V/1
  Bus Selector/1 -> override_notaus_gripper/1(u), override_notaus_purge/1(u), override_notaus/1(u)  "<ValvesOff>"
  off-mpye/1 -> Valves2Save9Analog/12
  purge-mpye/1 -> Valves2Save9Analog/11
  Valves2Save9Analog/10 -> final-u [-1..1]/1
  IOSetupBus/1 -> RT/1
  Valves2Save9Analog/1 -> Mux1/1
  Valves2Save9Analog/2 -> Mux1/2
  Valves2Save9Analog/3 -> Mux1/3
  Valves2Save9Analog/4 -> Mux1/4
  Valves2Save9Analog/5 -> Mux1/5
  Valves2Save9Analog/6 -> Mux1/6
  Valves2Save9Analog/7 -> Mux1/7
  Valves2Save9Analog/8 -> Mux1/8
  Valves2Save9Analog/9 -> Mux1/9
  Mux1/1 -> vProp/1
  Bus Selector3/9 -> Valves2Save9Analog/10  "<u-section3-bellows3>"
  Bus Selector3/8 -> Valves2Save9Analog/9  "<u-section3-bellows2>"
  Bus Selector3/7 -> Valves2Save9Analog/8  "<u-section3-bellows1>"
  Bus Selector3/6 -> Valves2Save9Analog/7  "<u-section2-bellows3>"
  Bus Selector3/5 -> Valves2Save9Analog/6  "<u-section2-bellows2>"
  Bus Selector3/4 -> Valves2Save9Analog/5  "<u-section2-bellows1>"
  Bus Selector3/3 -> Valves2Save9Analog/4  "<u-section1-bellows3>"
  Bus Selector3/2 -> Valves2Save9Analog/3  "<u-section1-bellows2>"
  Bus Selector3/1 -> Valves2Save9Analog/2  "<u-section1-bellows1>"
  Bus Selector4/1 -> Mux/1  "<up-section1-bellows1>"
  Bus Selector4/2 -> Mux/2  "<up-section1-bellows2>"
  Bus Selector4/3 -> Mux/3  "<up-section1-bellows3>"
  Bus Selector4/4 -> Mux/4  "<up-section2-bellows1>"
  Bus Selector4/5 -> Mux/5  "<up-section2-bellows2>"
  ControllerBus/1 -> Bus Selector4/1, Bus Selector1/1, Bus Selector3/1
  Bus Selector4/6 -> Mux/6  "<up-section2-bellows3>"
  Bus Selector4/7 -> Mux/7  "<up-section3-bellows1>"
  Bus Selector4/8 -> Mux/8  "<up-section3-bellows2>"
  Bus Selector4/9 -> Mux/9  "<up-section3-bellows3>"
  purge-digital/1 -> Valves2SaveXDigital_Purge/3
  off-digital/1 -> Valves2SaveXDigital_Purge/4
  Mux/1 -> Valves2SaveXDigital_Purge/2
  Valves2SaveXDigital_Purge/1 -> vSwitch/1
  Add1/1 -> Product1/1
  Bus Selector5/3 -> Product1/2  "<dac-2-scaling-factor-0-1>"
  Bus Selector5/2 -> Add1/2  "<dac-2-signal>"
  Bus Selector5/1 -> Add1/1  "<dac-2-add-offset-before-scaling>"
  Add2/1 -> Product2/1
  Bus Selector6/3 -> Product2/2  "<dac-3-scaling-factor-0-1>"
  Bus Selector6/2 -> Add2/2  "<dac-3-signal>"
  Bus Selector6/1 -> Add2/1  "<dac-3-add-offset-before-scaling>"
  toSiglabBus/1 -> Bus Selector2/1, Bus Selector5/1, Bus Selector6/1
  Product2/1 -> Mux2/3
  Product1/1 -> Mux2/2
  Product/1 -> Mux2/1
  Mux2/1 -> Saturation [0,1]/1
  Valves2SaveXDigital_Gripper/1 -> GripperOn/1
  gripper-purge-open/1 -> Valves2SaveXDigital_Gripper/3
  gripper-off-close/1 -> Valves2SaveXDigital_Gripper/4
  Bus Selector1/1 -> Valves2SaveXDigital_Gripper/2  "<Gripper>"
  override_notaus_purge/1(y) -> Valves2SaveXDigital_Purge/1
  override_notaus/1(y) -> Valves2Save9Analog/1
  override_notaus_gripper/1(y) -> Valves2SaveXDigital_Gripper/1

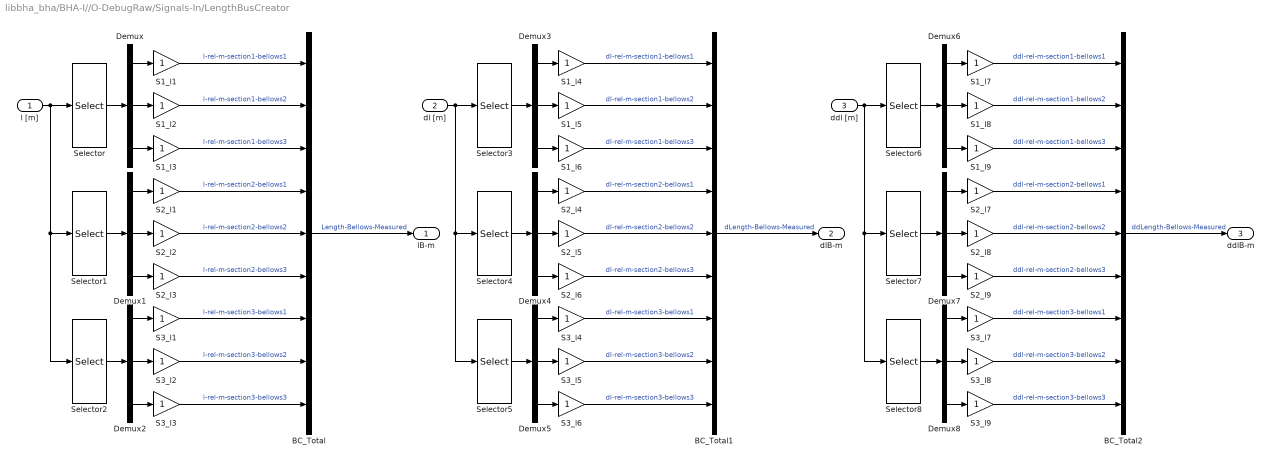
== system libbha_bha/BHA-I//O-DebugRaw/Signals-In/LengthBusCreator ==
  l [m] : Inport
  dl [m] : Inport  Port=2
  ddl [m] : Inport  Port=3
  BC_Total : BusCreator  Inputs=9
  BC_Total1 : BusCreator  Inputs=9
  BC_Total2 : BusCreator  Inputs=9
  Demux{,1..8} (9 alike) : Demux  Outputs=3
  S1_l{1..9} (9 alike) : Gain
  S2_l{1..9} (9 alike) : Gain
  S3_l{1..9} (9 alike) : Gain
  Selector : Selector  InputPortWidth=9  IndexOptions=Index vector (dialog)  Indices=[1 2 3]  OutputSizes=1
  Selector1 : Selector  InputPortWidth=9  IndexOptions=Index vector (dialog)  Indices=[4 5 6]  OutputSizes=1
  Selector2 : Selector  InputPortWidth=9  IndexOptions=Index vector (dialog)  Indices=[7 8 9]  OutputSizes=1
  Selector3 : Selector  InputPortWidth=9  IndexOptions=Index vector (dialog)  Indices=[1 2 3]  OutputSizes=1
  Selector4 : Selector  InputPortWidth=9  IndexOptions=Index vector (dialog)  Indices=[4 5 6]  OutputSizes=1
  Selector5 : Selector  InputPortWidth=9  IndexOptions=Index vector (dialog)  Indices=[7 8 9]  OutputSizes=1
  Selector6 : Selector  InputPortWidth=9  IndexOptions=Index vector (dialog)  Indices=[1 2 3]  OutputSizes=1
  Selector7 : Selector  InputPortWidth=9  IndexOptions=Index vector (dialog)  Indices=[4 5 6]  OutputSizes=1
  Selector8 : Selector  InputPortWidth=9  IndexOptions=Index vector (dialog)  Indices=[7 8 9]  OutputSizes=1
  lB-m : Outport
  dlB-m : Outport  Port=2
  ddlB-m : Outport  Port=3
  wires:
  BC_Total/1 -> lB-m/1  "Length-Bellows-Measured"
  S3_l1/1 -> BC_Total/7  "l-rel-m-section3-bellows1"
  S1_l2/1 -> BC_Total/2  "l-rel-m-section1-bellows2"
  S1_l3/1 -> BC_Total/3  "l-rel-m-section1-bellows3"
  S2_l1/1 -> BC_Total/4  "l-rel-m-section2-bellows1"
  S3_l2/1 -> BC_Total/8  "l-rel-m-section3-bellows2"
  S3_l3/1 -> BC_Total/9  "l-rel-m-section3-bellows3"
  S2_l2/1 -> BC_Total/5  "l-rel-m-section2-bellows2"
  S2_l3/1 -> BC_Total/6  "l-rel-m-section2-bellows3"
  S1_l1/1 -> BC_Total/1  "l-rel-m-section1-bellows1"
  Demux/1 -> S1_l1/1
  Demux/2 -> S1_l2/1
  Demux/3 -> S1_l3/1
  Demux1/2 -> S2_l2/1
  Demux1/1 -> S2_l1/1
  Demux1/3 -> S2_l3/1
  Demux2/1 -> S3_l1/1
  Demux2/2 -> S3_l2/1
  Demux2/3 -> S3_l3/1
  Selector/1 -> Demux/1
  Selector1/1 -> Demux1/1
  Selector2/1 -> Demux2/1
  l [m]/1 -> Selector2/1, Selector1/1, Selector/1
  BC_Total1/1 -> dlB-m/1  "dLength-Bellows-Measured"
  S3_l4/1 -> BC_Total1/7  "dl-rel-m-section3-bellows1"
  S1_l5/1 -> BC_Total1/2  "dl-rel-m-section1-bellows2"
  S1_l6/1 -> BC_Total1/3  "dl-rel-m-section1-bellows3"
  S2_l4/1 -> BC_Total1/4  "dl-rel-m-section2-bellows1"
  S3_l5/1 -> BC_Total1/8  "dl-rel-m-section3-bellows2"
  S3_l6/1 -> BC_Total1/9  "dl-rel-m-section3-bellows3"
  S2_l5/1 -> BC_Total1/5  "dl-rel-m-section2-bellows2"
  S2_l6/1 -> BC_Total1/6  "dl-rel-m-section2-bellows3"
  S1_l4/1 -> BC_Total1/1  "dl-rel-m-section1-bellows1"
  Demux3/1 -> S1_l4/1
  Demux3/2 -> S1_l5/1
  Demux3/3 -> S1_l6/1
  Demux4/2 -> S2_l5/1
  Demux4/1 -> S2_l4/1
  Demux4/3 -> S2_l6/1
  Demux5/1 -> S3_l4/1
  Demux5/2 -> S3_l5/1
  Demux5/3 -> S3_l6/1
  Selector3/1 -> Demux3/1
  Selector4/1 -> Demux4/1
  Selector5/1 -> Demux5/1
  dl [m]/1 -> Selector3/1, Selector4/1, Selector5/1
  BC_Total2/1 -> ddlB-m/1  "ddLength-Bellows-Measured"
  S3_l7/1 -> BC_Total2/7  "ddl-rel-m-section3-bellows1"
  S1_l8/1 -> BC_Total2/2  "ddl-rel-m-section1-bellows2"
  S1_l9/1 -> BC_Total2/3  "ddl-rel-m-section1-bellows3"
  S2_l7/1 -> BC_Total2/4  "ddl-rel-m-section2-bellows1"
  S3_l8/1 -> BC_Total2/8  "ddl-rel-m-section3-bellows2"
  S3_l9/1 -> BC_Total2/9  "ddl-rel-m-section3-bellows3"
  S2_l8/1 -> BC_Total2/5  "ddl-rel-m-section2-bellows2"
  S2_l9/1 -> BC_Total2/6  "ddl-rel-m-section2-bellows3"
  S1_l7/1 -> BC_Total2/1  "ddl-rel-m-section1-bellows1"
  Demux6/1 -> S1_l7/1
  Demux6/2 -> S1_l8/1
  Demux6/3 -> S1_l9/1
  Demux7/2 -> S2_l8/1
  Demux7/1 -> S2_l7/1
  Demux7/3 -> S2_l9/1
  Demux8/1 -> S3_l7/1
  Demux8/2 -> S3_l8/1
  Demux8/3 -> S3_l9/1
  Selector6/1 -> Demux6/1
  Selector7/1 -> Demux7/1
  Selector8/1 -> Demux8/1
  ddl [m]/1 -> Selector8/1, Selector7/1, Selector6/1

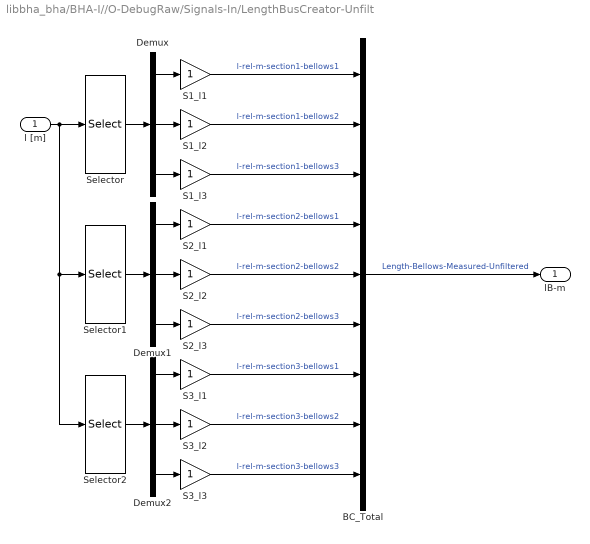
== system libbha_bha/BHA-I//O-DebugRaw/Signals-In/LengthBusCreator-Unfilt ==
  l [m] : Inport
  BC_Total : BusCreator  Inputs=9
  Demux : Demux  Outputs=3
  Demux1 : Demux  Outputs=3
  Demux2 : Demux  Outputs=3
  S1_l1 : Gain
  S1_l2 : Gain
  S1_l3 : Gain
  S2_l1 : Gain
  S2_l2 : Gain
  S2_l3 : Gain
  S3_l1 : Gain
  S3_l2 : Gain
  S3_l3 : Gain
  Selector : Selector  InputPortWidth=9  IndexOptions=Index vector (dialog)  Indices=[1 2 3]  OutputSizes=1
  Selector1 : Selector  InputPortWidth=9  IndexOptions=Index vector (dialog)  Indices=[4 5 6]  OutputSizes=1
  Selector2 : Selector  InputPortWidth=9  IndexOptions=Index vector (dialog)  Indices=[7 8 9]  OutputSizes=1
  lB-m : Outport
  wires:
  l [m]/1 -> Selector/1, Selector1/1, Selector2/1
  Selector2/1 -> Demux2/1
  Selector1/1 -> Demux1/1
  Selector/1 -> Demux/1
  Demux2/3 -> S3_l3/1
  Demux2/2 -> S3_l2/1
  Demux2/1 -> S3_l1/1
  Demux1/3 -> S2_l3/1
  Demux1/1 -> S2_l1/1
  Demux1/2 -> S2_l2/1
  Demux/3 -> S1_l3/1
  Demux/2 -> S1_l2/1
  Demux/1 -> S1_l1/1
  S1_l1/1 -> BC_Total/1  "l-rel-m-section1-bellows1"
  S2_l3/1 -> BC_Total/6  "l-rel-m-section2-bellows3"
  S2_l2/1 -> BC_Total/5  "l-rel-m-section2-bellows2"
  S3_l3/1 -> BC_Total/9  "l-rel-m-section3-bellows3"
  S3_l2/1 -> BC_Total/8  "l-rel-m-section3-bellows2"
  S2_l1/1 -> BC_Total/4  "l-rel-m-section2-bellows1"
  S1_l3/1 -> BC_Total/3  "l-rel-m-section1-bellows3"
  S1_l2/1 -> BC_Total/2  "l-rel-m-section1-bellows2"
  S3_l1/1 -> BC_Total/7  "l-rel-m-section3-bellows1"
  BC_Total/1 -> lB-m/1  "Length-Bellows-Measured-Unfiltered"

== system libbha_bha/BHA-I//O-DebugRaw/Signals-In/LengthRematch2Rel ==
  "l-mess [m] " : Inport
  Demux : Demux  Outputs=9
  Mux : Mux  Inputs=9
  Sum{,1..5} (6 alike) : Sum  Inputs=-+|
  l-delta [m] : Outport
  wires:
  Mux/1 -> l-delta [m]/1
  "l-mess [m] "/1 -> Demux/1
  Demux/1 -> Sum/1, Mux/1  "Bellows1"
  Demux/2 -> Sum1/1, Mux/2  "Bellows2"
  Demux/3 -> Sum2/1, Mux/3  "Bellows3"
  Demux/4 -> Sum/2, Sum3/1
  Demux/5 -> Sum1/2, Sum4/1
  Demux/6 -> Sum2/2, Sum5/1
  Demux/7 -> Sum3/2
  Demux/8 -> Sum4/2
  Demux/9 -> Sum5/2
  Sum/1 -> Mux/4  "Bellows1"
  Sum1/1 -> Mux/5  "Bellows2"
  Sum2/1 -> Mux/6  "Bellows3"
  Sum3/1 -> Mux/7  "Bellows1"
  Sum4/1 -> Mux/8  "Bellows2"
  Sum5/1 -> Mux/9  "Bellows3"

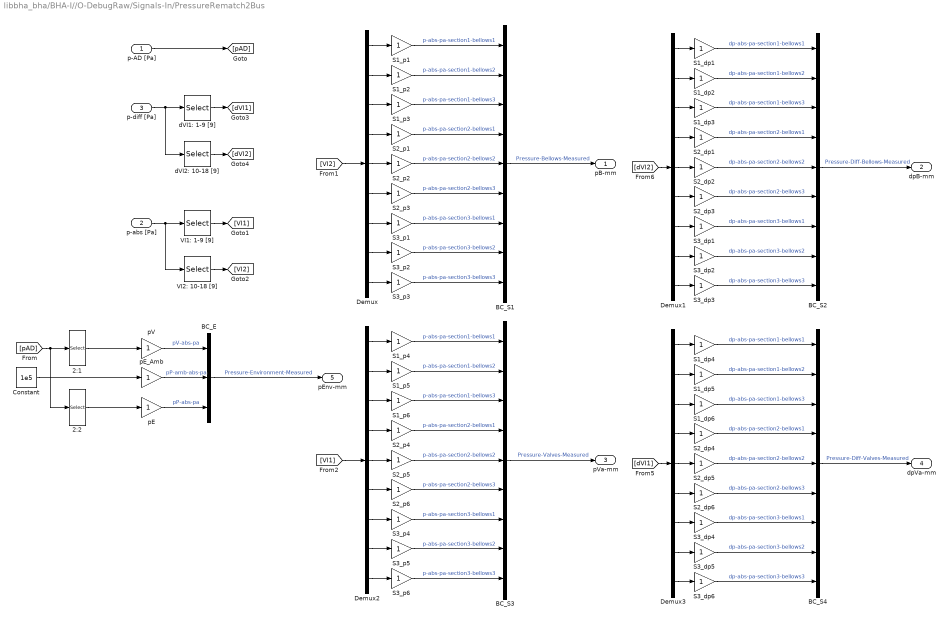
== system libbha_bha/BHA-I//O-DebugRaw/Signals-In/PressureRematch2Bus ==
  p-AD [Pa] : Inport  PortDimensions=2
      settings: AttributesFormatString=2 Signals
  p-abs [Pa] : Inport  Port=2  PortDimensions=18
      settings: AttributesFormatString=18 Signals
  p-diff [Pa] : Inport  Port=3  PortDimensions=18
      settings: AttributesFormatString=18 Signals
  2:1 : Selector  InputPortWidth=2  IndexOptions=Index vector (dialog)  Indices=1  OutputSizes=1
  2:2 : Selector  InputPortWidth=2  IndexOptions=Index vector (dialog)  Indices=2  OutputSizes=1
  BC_E : BusCreator  Inputs=3
  BC_S{1..4} (4 alike) : BusCreator  Inputs=9
  Constant : Constant  Value=1e5
  Demux{,1..3} (4 alike) : Demux  Outputs=9
  S1_dp{1..6} (6 alike) : Gain
  S1_p{1..6} (6 alike) : Gain
  S2_dp{1..6} (6 alike) : Gain
  S2_p{1..6} (6 alike) : Gain
  S3_dp{1..6} (6 alike) : Gain
  S3_p{1..6} (6 alike) : Gain
  VI1: 1-9 [9] : Selector  InputPortWidth=18  IndexOptions=Starting index (dialog)  Indices=1  OutputSizes=9
  VI2: 10-18 [9] : Selector  InputPortWidth=18  IndexOptions=Starting index (dialog)  Indices=10  OutputSizes=9
  dVI1: 1-9 [9] : Selector  InputPortWidth=18  IndexOptions=Starting index (dialog)  Indices=1  OutputSizes=9
  dVI2: 10-18 [9] : Selector  InputPortWidth=18  IndexOptions=Starting index (dialog)  Indices=10  OutputSizes=9
  pE : Gain
  pE_Amb : Gain
  pV : Gain
  pB-mm : Outport
  dpB-mm : Outport  Port=2
  pVa-mm : Outport  Port=3
  dpVa-mm : Outport  Port=4
  pEnv-mm : Outport  Port=5
  wires:
  pE_Amb/1 -> BC_E/2  "pP-amb-abs-pa"
  pE/1 -> BC_E/3  "pP-abs-pa"
  pV/1 -> BC_E/1  "pV-abs-pa"
  S3_p3/1 -> BC_S1/9  "p-abs-pa-section3-bellows3"
  S3_p2/1 -> BC_S1/8  "p-abs-pa-section3-bellows2"
  S3_p1/1 -> BC_S1/7  "p-abs-pa-section3-bellows1"
  S2_p3/1 -> BC_S1/6  "p-abs-pa-section2-bellows3"
  S2_p2/1 -> BC_S1/5  "p-abs-pa-section2-bellows2"
  S2_p1/1 -> BC_S1/4  "p-abs-pa-section2-bellows1"
  BC_E/1 -> pEnv-mm/1  "Pressure-Environment-Measured"
  BC_S1/1 -> pB-mm/1  "Pressure-Bellows-Measured"
  S1_p3/1 -> BC_S1/3  "p-abs-pa-section1-bellows3"
  S1_p2/1 -> BC_S1/2  "p-abs-pa-section1-bellows2"
  S1_p1/1 -> BC_S1/1  "p-abs-pa-section1-bellows1"
  p-AD [Pa]/1 -> [pAD]
  VI2: 10-18 [9]/1 -> [VI2]
  VI1: 1-9 [9]/1 -> [VI1]
  [VI2] -> Demux/1
  Constant/1 -> pE_Amb/1
  2:2/1 -> pE/1
  dVI2: 10-18 [9]/1 -> [dVI2]
  dVI1: 1-9 [9]/1 -> [dVI1]
  p-diff [Pa]/1 -> dVI2: 10-18 [9]/1, dVI1: 1-9 [9]/1
  S3_dp3/1 -> BC_S2/9  "dp-abs-pa-section3-bellows3"
  S3_dp2/1 -> BC_S2/8  "dp-abs-pa-section3-bellows2"
  S3_dp1/1 -> BC_S2/7  "dp-abs-pa-section3-bellows1"
  S2_dp3/1 -> BC_S2/6  "dp-abs-pa-section2-bellows3"
  S2_dp2/1 -> BC_S2/5  "dp-abs-pa-section2-bellows2"
  S2_dp1/1 -> BC_S2/4  "dp-abs-pa-section2-bellows1"
  S1_dp3/1 -> BC_S2/3  "dp-abs-pa-section1-bellows3"
  S1_dp2/1 -> BC_S2/2  "dp-abs-pa-section1-bellows2"
  S1_dp1/1 -> BC_S2/1  "dp-abs-pa-section1-bellows1"
  BC_S2/1 -> dpB-mm/1  "Pressure-Diff-Bellows-Measured"
  p-abs [Pa]/1 -> VI2: 10-18 [9]/1, VI1: 1-9 [9]/1
  2:1/1 -> pV/1
  [pAD] -> 2:2/1, 2:1/1
  Demux/6 -> S2_p3/1
  Demux/7 -> S3_p1/1
  Demux/5 -> S2_p2/1
  Demux/4 -> S2_p1/1
  Demux/8 -> S3_p2/1
  Demux/9 -> S3_p3/1
  Demux/3 -> S1_p3/1
  Demux/2 -> S1_p2/1
  Demux/1 -> S1_p1/1
  Demux1/4 -> S2_dp1/1
  Demux1/6 -> S2_dp3/1
  Demux1/8 -> S3_dp2/1
  Demux1/9 -> S3_dp3/1
  Demux1/1 -> S1_dp1/1
  Demux1/3 -> S1_dp3/1
  Demux1/2 -> S1_dp2/1
  Demux1/7 -> S3_dp1/1
  Demux1/5 -> S2_dp2/1
  S3_p6/1 -> BC_S3/9  "p-abs-pa-section3-bellows3"
  S3_p5/1 -> BC_S3/8  "p-abs-pa-section3-bellows2"
  S3_p4/1 -> BC_S3/7  "p-abs-pa-section3-bellows1"
  S2_p6/1 -> BC_S3/6  "p-abs-pa-section2-bellows3"
  S2_p5/1 -> BC_S3/5  "p-abs-pa-section2-bellows2"
  S2_p4/1 -> BC_S3/4  "p-abs-pa-section2-bellows1"
  BC_S3/1 -> pVa-mm/1  "Pressure-Valves-Measured"
  S1_p6/1 -> BC_S3/3  "p-abs-pa-section1-bellows3"
  S1_p5/1 -> BC_S3/2  "p-abs-pa-section1-bellows2"
  S1_p4/1 -> BC_S3/1  "p-abs-pa-section1-bellows1"
  [VI1] -> Demux2/1
  S3_dp6/1 -> BC_S4/9  "dp-abs-pa-section3-bellows3"
  S3_dp5/1 -> BC_S4/8  "dp-abs-pa-section3-bellows2"
  S3_dp4/1 -> BC_S4/7  "dp-abs-pa-section3-bellows1"
  S2_dp6/1 -> BC_S4/6  "dp-abs-pa-section2-bellows3"
  S2_dp5/1 -> BC_S4/5  "dp-abs-pa-section2-bellows2"
  S2_dp4/1 -> BC_S4/4  "dp-abs-pa-section2-bellows1"
  S1_dp6/1 -> BC_S4/3  "dp-abs-pa-section1-bellows3"
  S1_dp5/1 -> BC_S4/2  "dp-abs-pa-section1-bellows2"
  S1_dp4/1 -> BC_S4/1  "dp-abs-pa-section1-bellows1"
  BC_S4/1 -> dpVa-mm/1  "Pressure-Diff-Valves-Measured"
  Demux2/6 -> S2_p6/1
  Demux2/7 -> S3_p4/1
  Demux2/5 -> S2_p5/1
  Demux2/4 -> S2_p4/1
  Demux2/8 -> S3_p5/1
  Demux2/9 -> S3_p6/1
  Demux2/3 -> S1_p6/1
  Demux2/2 -> S1_p5/1
  Demux2/1 -> S1_p4/1
  Demux3/4 -> S2_dp4/1
  Demux3/6 -> S2_dp6/1
  Demux3/8 -> S3_dp5/1
  Demux3/9 -> S3_dp6/1
  Demux3/1 -> S1_dp4/1
  Demux3/3 -> S1_dp6/1
  Demux3/2 -> S1_dp5/1
  Demux3/7 -> S3_dp4/1
  Demux3/5 -> S2_dp5/1
  [dVI2] -> Demux1/1
  [dVI1] -> Demux3/1

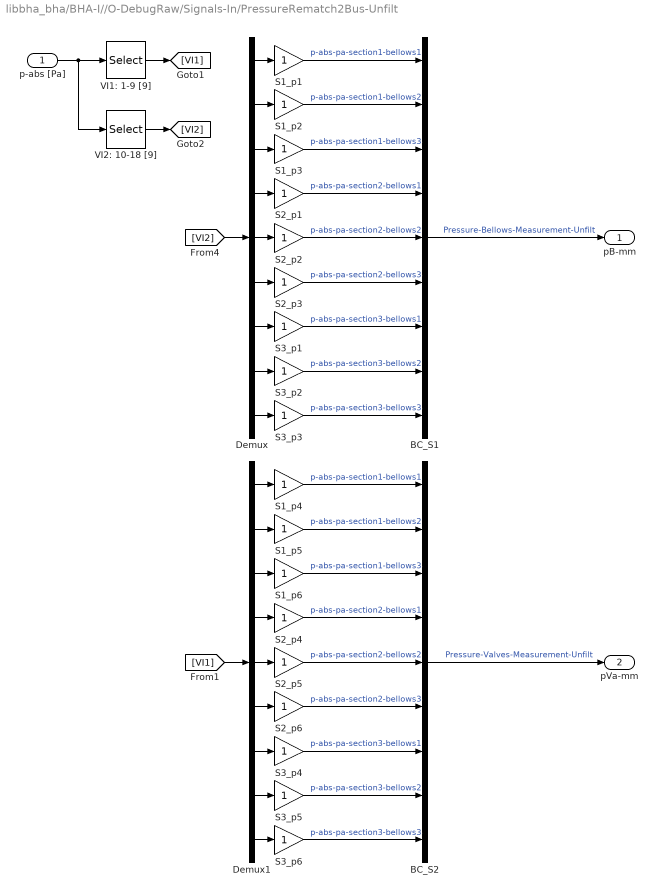
== system libbha_bha/BHA-I//O-DebugRaw/Signals-In/PressureRematch2Bus-Unfilt ==
  p-abs [Pa] : Inport  PortDimensions=18
      settings: AttributesFormatString=18 Signals
  BC_S1 : BusCreator  Inputs=9
  BC_S2 : BusCreator  Inputs=9
  Demux : Demux  Outputs=9
  Demux1 : Demux  Outputs=9
  S1_p{1..6} (6 alike) : Gain
  S2_p{1..6} (6 alike) : Gain
  S3_p{1..6} (6 alike) : Gain
  VI1: 1-9 [9] : Selector  InputPortWidth=18  IndexOptions=Starting index (dialog)  Indices=1  OutputSizes=9
  VI2: 10-18 [9] : Selector  InputPortWidth=18  IndexOptions=Starting index (dialog)  Indices=10  OutputSizes=9
  pB-mm : Outport
  pVa-mm : Outport  Port=2
  wires:
  p-abs [Pa]/1 -> VI1: 1-9 [9]/1, VI2: 10-18 [9]/1
  VI1: 1-9 [9]/1 -> [VI1]
  VI2: 10-18 [9]/1 -> [VI2]
  S1_p1/1 -> BC_S1/1  "p-abs-pa-section1-bellows1"
  S1_p2/1 -> BC_S1/2  "p-abs-pa-section1-bellows2"
  S1_p3/1 -> BC_S1/3  "p-abs-pa-section1-bellows3"
  BC_S1/1 -> pB-mm/1  "Pressure-Bellows-Measurement-Unfilt"
  S2_p1/1 -> BC_S1/4  "p-abs-pa-section2-bellows1"
  S2_p2/1 -> BC_S1/5  "p-abs-pa-section2-bellows2"
  S2_p3/1 -> BC_S1/6  "p-abs-pa-section2-bellows3"
  S3_p1/1 -> BC_S1/7  "p-abs-pa-section3-bellows1"
  S3_p2/1 -> BC_S1/8  "p-abs-pa-section3-bellows2"
  S3_p3/1 -> BC_S1/9  "p-abs-pa-section3-bellows3"
  Demux/2 -> S1_p2/1
  Demux/3 -> S1_p3/1
  Demux/1 -> S1_p1/1
  Demux/4 -> S2_p1/1
  Demux/5 -> S2_p2/1
  Demux/6 -> S2_p3/1
  Demux/7 -> S3_p1/1
  Demux/8 -> S3_p2/1
  Demux/9 -> S3_p3/1
  [VI2] -> Demux/1
  S1_p4/1 -> BC_S2/1  "p-abs-pa-section1-bellows1"
  S1_p5/1 -> BC_S2/2  "p-abs-pa-section1-bellows2"
  S1_p6/1 -> BC_S2/3  "p-abs-pa-section1-bellows3"
  BC_S2/1 -> pVa-mm/1  "Pressure-Valves-Measurement-Unfilt"
  S2_p4/1 -> BC_S2/4  "p-abs-pa-section2-bellows1"
  S2_p5/1 -> BC_S2/5  "p-abs-pa-section2-bellows2"
  S2_p6/1 -> BC_S2/6  "p-abs-pa-section2-bellows3"
  S3_p4/1 -> BC_S2/7  "p-abs-pa-section3-bellows1"
  S3_p5/1 -> BC_S2/8  "p-abs-pa-section3-bellows2"
  S3_p6/1 -> BC_S2/9  "p-abs-pa-section3-bellows3"
  Demux1/2 -> S1_p5/1
  Demux1/3 -> S1_p6/1
  Demux1/1 -> S1_p4/1
  Demux1/4 -> S2_p4/1
  Demux1/5 -> S2_p5/1
  Demux1/6 -> S2_p6/1
  Demux1/7 -> S3_p4/1
  Demux1/8 -> S3_p5/1
  Demux1/9 -> S3_p6/1
  [VI1] -> Demux1/1

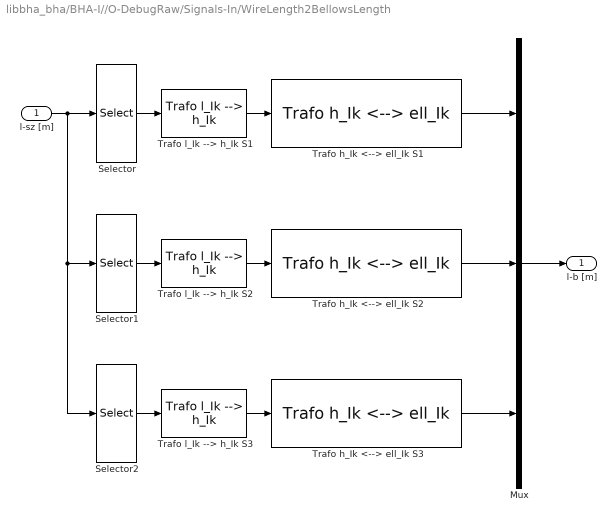
== system libbha_bha/BHA-I//O-DebugRaw/Signals-In/WireLength2BellowsLength ==
  l-sz [m] : Inport
  Mux : Mux  Inputs=3
  Selector : Selector  InputPortWidth=9  IndexOptions=Index vector (dialog)  Indices=[1 2 3]  OutputSizes=1
  Selector1 : Selector  InputPortWidth=9  IndexOptions=Index vector (dialog)  Indices=[4 5 6]  OutputSizes=1
  Selector2 : Selector  InputPortWidth=9  IndexOptions=Index vector (dialog)  Indices=[7 8 9]  OutputSizes=1
  Trafo h_Ik <--> ell_Ik S1 : libbha_kinematic_tools/Trafo h_Ik <--> ell_Ik  inv=off  ii=1  m_i=BHA.Trunk.vc.num_segm  r_Si=BHA.Trunk.r_ms_i  r_Ai=BHA.Trunk.r_mb_i
      settings: AttributesFormatString=Seilzughöhe <> Balgbogenlänge\ninv = %<inv> | Sektion %<ii>
  Trafo h_Ik <--> ell_Ik S2 : libbha_kinematic_tools/Trafo h_Ik <--> ell_Ik  inv=off  ii=2  m_i=BHA.Trunk.vc.num_segm  r_Si=BHA.Trunk.r_ms_i  r_Ai=BHA.Trunk.r_mb_i
      settings: AttributesFormatString=Seilzughöhe <> Balgbogenlänge\ninv = %<inv> | Sektion %<ii>
  Trafo h_Ik <--> ell_Ik S3 : libbha_kinematic_tools/Trafo h_Ik <--> ell_Ik  inv=off  ii=3  m_i=BHA.Trunk.vc.num_segm  r_Si=BHA.Trunk.r_ms_i  r_Ai=BHA.Trunk.r_mb_i
      settings: AttributesFormatString=Seilzughöhe <> Balgbogenlänge\ninv = %<inv> | Sektion %<ii>
  Trafo l_Ik --> h_Ik S1 : libbha_kinematic_tools/Trafo l_Ik --> h_Ik  ii=1 = gross
      settings: AttributesFormatString=Seilzuglänge > Seilzughöhe\nSektion %<ii>
  Trafo l_Ik --> h_Ik S2 : libbha_kinematic_tools/Trafo l_Ik --> h_Ik  ii=2 = mittel
      settings: AttributesFormatString=Seilzuglänge > Seilzughöhe\nSektion %<ii>
  Trafo l_Ik --> h_Ik S3 : libbha_kinematic_tools/Trafo l_Ik --> h_Ik  ii=3 = klein
      settings: AttributesFormatString=Seilzuglänge > Seilzughöhe\nSektion %<ii>
  l-b [m] : Outport
  wires:
  Mux/1 -> l-b [m]/1
  Trafo h_Ik <--> ell_Ik S3/1 -> Mux/3
  Trafo h_Ik <--> ell_Ik S1/1 -> Mux/1
  Trafo h_Ik <--> ell_Ik S2/1 -> Mux/2
  l-sz [m]/1 -> Selector/1, Selector1/1, Selector2/1
  Selector1/1 -> Trafo l_Ik --> h_Ik S2/1
  Selector2/1 -> Trafo l_Ik --> h_Ik S3/1
  Selector/1 -> Trafo l_Ik --> h_Ik S1/1
  Trafo l_Ik --> h_Ik S1/1 -> Trafo h_Ik <--> ell_Ik S1/1
  Trafo l_Ik --> h_Ik S2/1 -> Trafo h_Ik <--> ell_Ik S2/1
  Trafo l_Ik --> h_Ik S3/1 -> Trafo h_Ik <--> ell_Ik S3/1

== matlab function libbha_bha/BHA-I//O-DebugRaw/Signals-In/Honeywell Scaling ==
  data: U2p output; Vsupply input; Pmax input; Pmin input; offset_p output
function [U2p, offset_p] = hnwl(Vsupply, Pmax, Pmin)
%#codegen

%% Herleitung der Formel 
% Vgen = 0.8*Vsupply*(p-pmin)/(pmax-pmin) + 0.1*Vsupply
% -->
% p = (Vgen_mm - 0.1*Vsupply)/(0.8*Vsupply)*(pmax-pmin) + pmin

%% Umsetzung

U2p = (Pmax-Pmin)/(0.8*Vsupply);
offset_p = 0.1/0.8*(Pmax-Pmin) - Pmin;

%% Anwendung

% p_bar = V_mm * U2p - offset_p;

== matlab function libbha_bha/BHA-I//O-DebugRaw/Signals-Out/override_notaus_purge ==
  data: u input; y output
function y = notaus_rules(u)
%#codegen

    % Auswertung (Ausgang):
    %    1: Entlüften (Vakuum)
    %    2: Entlüften (Umgebung)

    switch u
        case 1 % Entlüften
            y = 2;
        case 2 % Zu (Block)
            y = 2;
        case 3 % Vakuum
            y = 1;
        otherwise
            y = 0;
    end

end

== matlab function libbha_bha/BHA-I//O-DebugRaw/Signals-Out/override_notaus ==
  data: u input; y output
function y = notaus_rules(u)
%#codegen

    % Auswertung (Ausgang):
    %    1: Entlüften
    %    2: Block

    switch u
        case 1 % Entlüften
            y = 1;
        case 2 % Zu (Block)
            y = 2;
        case 3 % Vakuum
            y = 1;
        otherwise
            y = 0;
    end

end

== matlab function libbha_bha/BHA-I//O-DebugRaw/Signals-Out/override_notaus_gripper ==
  data: u input; y output
function y = notaus_rules(u)
%#codegen

    % Auswertung (Ausgang):
    %    1: Auf
    %    2: Zu

    switch u
        case 1 % Entlüften
            y = 1;
        case 2 % Zu (Block)
            y = 2;
        case 3 % Vakuum
            y = 1;
        otherwise
            y = 0;
    end

end
